simulink model "Qn2"  (R2022b)
settings: Solver=VariableStepAuto  StartTime=0.0  StopTime=10.0  MaxStep=0.01  RelTol=1e-3
settings Model: Creator=nmary  LastModifiedBy=nmary

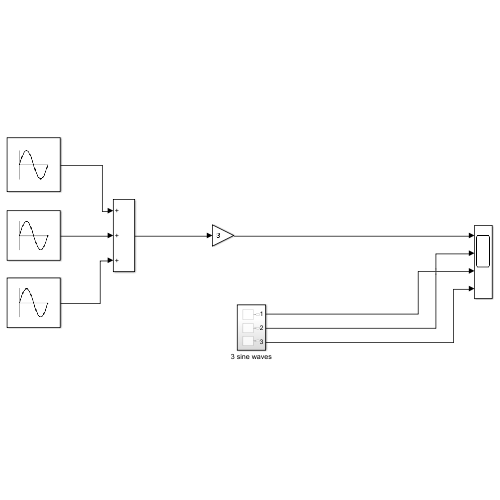
[thumbnail: Simulink's stored preview of the top-level diagram]
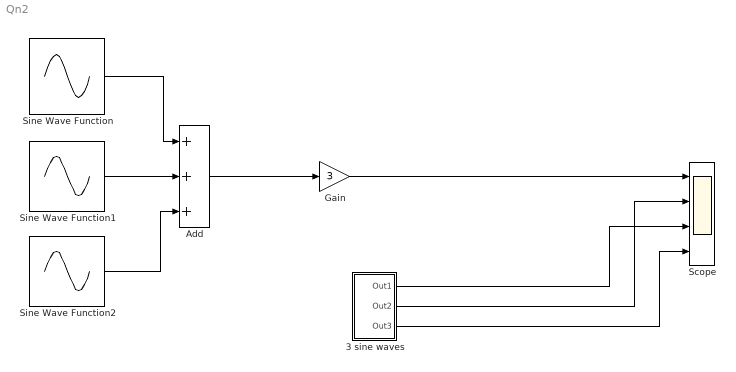
== system Qn2 ==
  3 sine waves : Subsystem
  Add : Sum  Inputs=+++
  Gain : Gain  Gain=3
  Scope : Scope  NumInputPorts=4
  Sine Wave Function : Sin  Frequency=5  SampleTime=0
  Sine Wave Function1 : Sin  Frequency=8  SampleTime=0
  Sine Wave Function2 : Sin  Frequency=10  SampleTime=0
  wires:
  Sine Wave Function/1 -> Add/1
  Sine Wave Function1/1 -> Add/2
  Sine Wave Function2/1 -> Add/3
  Add/1 -> Gain/1
  3 sine waves/2(Out2) -> Scope/2
  3 sine waves/1(Out1) -> Scope/3
  3 sine waves/3(Out3) -> Scope/4
  Gain/1 -> Scope/1

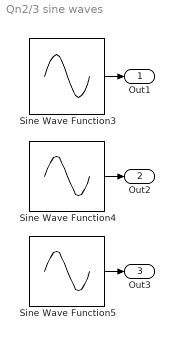
== system Qn2/3 sine waves ==
  Sine Wave Function3 : Sin  Frequency=5  SampleTime=0
  Sine Wave Function4 : Sin  Frequency=8  SampleTime=0
  Sine Wave Function5 : Sin  Frequency=10  SampleTime=0
  Out1 : Outport
  Out2 : Outport  Port=2
  Out3 : Outport  Port=3
  wires:
  Sine Wave Function4/1 -> Out2/1
  Sine Wave Function3/1 -> Out1/1
  Sine Wave Function5/1 -> Out3/1
